simulink model "geodetic_position_calculate"  (R2024b)
settings: Solver=VariableStepAuto  StartTime=0.0  StopTime=10.0  RelTol=1e-3
settings Model: Creator=satvik_sh  LastModifiedBy=satvik_sh

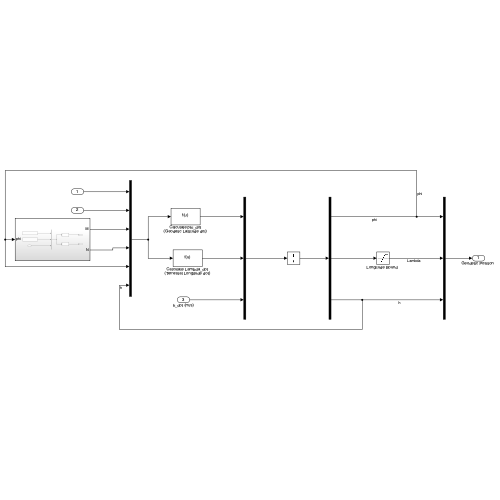
[thumbnail: Simulink's stored preview of the top-level diagram]
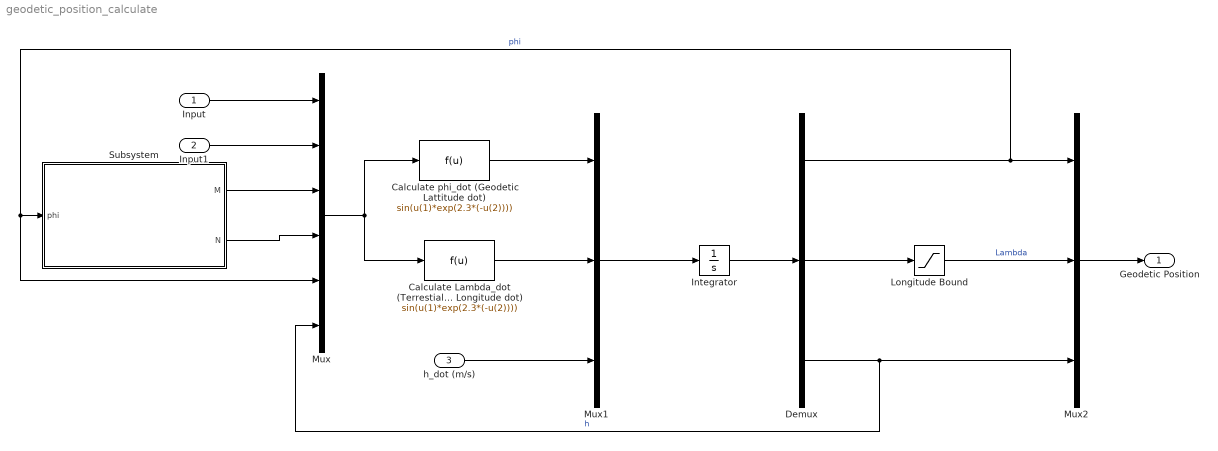
== system geodetic_position_calculate ==
  Input : Inport
  Input1 : Inport  Port=2
  h_dot (m/s) : Inport  Port=3
  Calculate Lambda_dot (Terrestial Longitude dot) : Fcn  Expr=sin(u(1)*exp(2.3*(-u(2))))
  "Calculate phi_dot (Geodetic Lattitude dot) " : Fcn  Expr=sin(u(1)*exp(2.3*(-u(2))))
  Demux : Demux  Outputs=3
  Integrator : Integrator
  "Longitude Bound " : Saturate  UpperLimit=pi  LowerLimit=-pi
  Mux : Mux  Inputs=6
  Mux1 : Mux  Inputs=3
  Mux2 : Mux  Inputs=3
  Subsystem : Subsystem
  "Geodetic Position " : Outport
  wires:
  h_dot (m/s)/1 -> Mux1/3
  Input/1 -> Mux/1
  Input1/1 -> Mux/2
  Mux1/1 -> Integrator/1
  "Calculate phi_dot (Geodetic Lattitude dot) "/1 -> Mux1/1
  Calculate Lambda_dot (Terrestial Longitude dot)/1 -> Mux1/2
  Integrator/1 -> Demux/1
  Mux/1 -> Calculate Lambda_dot (Terrestial Longitude dot)/1, "Calculate phi_dot (Geodetic Lattitude dot) "/1
  Demux/1 -> Mux/5, Subsystem/1(phi), Mux2/1  "phi"
  Demux/3 -> Mux/6, Mux2/3  "h"
  Demux/2 -> "Longitude Bound "/1
  "Longitude Bound "/1 -> Mux2/2  "Lambda"
  Mux2/1 -> "Geodetic Position "/1
  Subsystem/1(M) -> Mux/3
  Subsystem/2(N) -> Mux/4

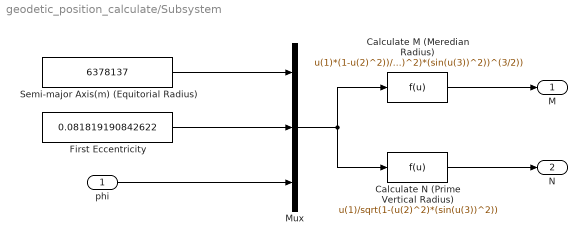
== system geodetic_position_calculate/Subsystem ==
  phi : Inport
  "Calculate M (Meredian Radius) " : Fcn  Expr=u(1)*(1-u(2)^2))/((1-u(2)^2)*(sin(u(3))^2))^(3/2))
  Calculate N (Prime Vertical Radius) : Fcn  Expr=u(1)/sqrt(1-(u(2)^2)*(sin(u(3))^2))
  First Eccentricity : Constant  Value=0.081819190842622
  Mux : Mux  Inputs=3
  Semi-major Axis(m) (Equitorial Radius) : Constant  Value=6378137
  M : Outport
  N : Outport  Port=2
  wires:
  First Eccentricity/1 -> Mux/2
  phi/1 -> Mux/3
  Calculate N (Prime Vertical Radius)/1 -> N/1
  Mux/1 -> Calculate N (Prime Vertical Radius)/1, "Calculate M (Meredian Radius) "/1
  "Calculate M (Meredian Radius) "/1 -> M/1
  Semi-major Axis(m) (Equitorial Radius)/1 -> Mux/1
